simulink model "zad2disc"  (R2014b)
settings: Solver=ode45  StartTime=0.0  StopTime=70  RelTol=1e-3
values from neighbouring files (symbols this model uses):
  Tp = 1    [zad10.m]    (also in zad11.m; zad3.m = Tp_vect(i); zad9.m)
undefined symbols (not defined in the file or in its folder): a1, a2, a3, a4, K, T1, T2
settings Model: Creator=kuba  LastModifiedBy=kuba

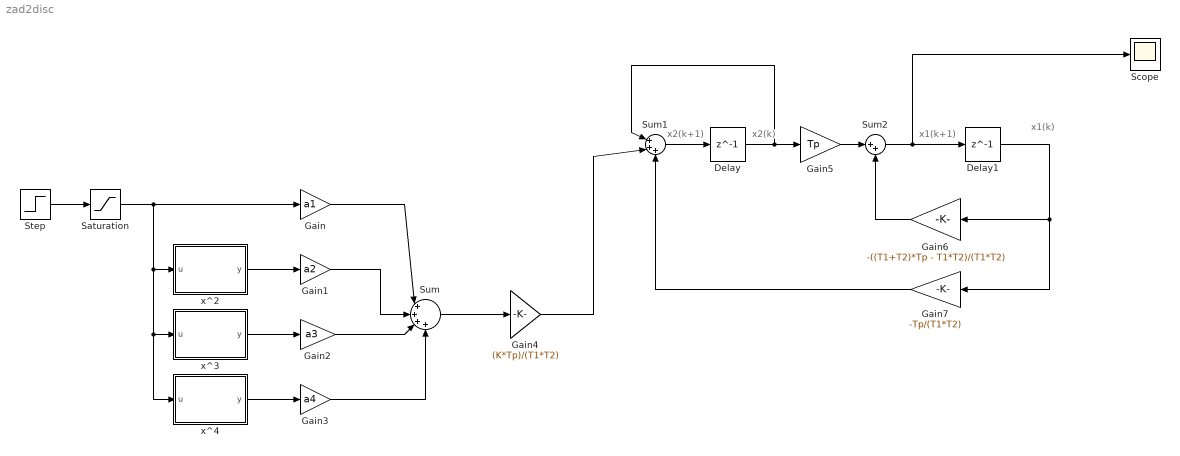
== system zad2disc ==
  note: x2(k+1)
  note: x1(k+1)
  note: x2(k)
  note: x1(k)
  Delay : Delay  DelayLength=1  InitialCondition=0  SampleTime=Tp
  Delay1 : Delay  DelayLength=1  InitialCondition=0  SampleTime=Tp
  Gain : Gain  Gain=a1  SampleTime=Tp
  Gain1 : Gain  Gain=a2  SampleTime=Tp
  Gain2 : Gain  Gain=a3  SampleTime=Tp
  Gain3 : Gain  Gain=a4  SampleTime=Tp
  Gain4 : Gain  Gain=(K*Tp)/(T1*T2)
  Gain5 : Gain  Gain=Tp
  Gain6 : Gain  Gain=-((T1+T2)*Tp - T1*T2)/(T1*T2)
  Gain7 : Gain  Gain=-Tp/(T1*T2)
  Saturation : Saturate  UpperLimit=1  LowerLimit=-1
  Scope : Scope
      settings: TimeRange=100  YMin=-1  YMax=1
  Step : Step  SampleTime=0
  Sum : Sum  Inputs=|++++
  Sum1 : Sum  Inputs=|+++
  Sum2 : Sum  Inputs=|++
  x^2 : MATLAB Function  TreatAsAtomicUnit=on
  x^3 : MATLAB Function  TreatAsAtomicUnit=on
  x^4 : MATLAB Function  TreatAsAtomicUnit=on
  wires:
  Saturation/1 -> x^4/1(u), x^3/1(u), x^2/1(u), Gain/1
  x^2/1(y) -> Gain1/1
  x^3/1(y) -> Gain2/1
  x^4/1(y) -> Gain3/1
  Gain/1 -> Sum/1
  Gain1/1 -> Sum/2
  Gain2/1 -> Sum/3
  Gain3/1 -> Sum/4
  Sum/1 -> Gain4/1
  Step/1 -> Saturation/1
  Gain4/1 -> Sum1/2
  Sum1/1 -> Delay/1
  Delay/1 -> Gain5/1, Sum1/1
  Gain5/1 -> Sum2/1
  Sum2/1 -> Scope/1, Delay1/1
  Gain6/1 -> Sum2/2
  Gain7/1 -> Sum1/3
  Delay1/1 -> Gain7/1, Gain6/1

== matlab function zad2disc/x^3 ==
  data: u input; y output
function y = cube(u)
y = u^3;

== matlab function zad2disc/x^2 ==
  data: u input; y output
function y = square(u)
y = u^2;

== matlab function zad2disc/x^4 ==
  data: u input; y output
function y = quad(u)
y = u^4;
